simulink model "satellite2"  (R2025b)
settings: Solver=FixedStepAuto  StartTime=0.0  StopTime=5000  FixedStep=dt  MinStep=0.0001  RelTol=1e-3
values from neighbouring files (symbols this model uses):
  A_mw = [ ... (first row only)    [init_params.m]
  A_w = [ ... (first row only)    [init_params.m]
  alpha1 = 0.1    [init_params.m]
  alpha2 = 0.1    [init_params.m]
  angle0 = eAR'    [init_params.m]
  area_d = 4    [init_params.m]
  area_m2 = 0.0127    [init_params.m]
  area_s = 2    [init_params.m]
  ARW_deg_per_sqrt_h = 0.01    [init_params.m]
  B_mw = [ ... (first row only)    [init_params.m]
  beta1 = 0.01    [init_params.m]
  beta2 = 0.01    [init_params.m]
  bias0_deg_h = 0.01    [init_params.m]
  C_bus = 0.001    [init_params.m]
  C_mw = [ ... (first row only)    [init_params.m]
  Cd = 2.2    [init_params.m]
  cos_g_max = cos(gamma_max)    [init_params.m]
  Cr = 1.2    [init_params.m]
  D_max = 1    [init_params.m]
  Delta_D = 0.001    [init_params.m]
  dP_th = 0.05    [init_params.m]
  epsilon = 0.01    [init_params.m]
  eta = 0.7    [init_params.m]
  eta_buck = 0.9    [init_params.m]
  eta_chg = 0.95    [init_params.m]
  f = 2.2e9    (= 2200000000)    [init_params.m]
  f_n_hz = 400    [init_params.m]
  g0 = 9.80665    [init_params.m]
  G0 = 1366.1    [init_params.m]
  Gr_dB = 20    [init_params.m]
  Gt_dB = 3    [init_params.m]
  H = 50e3    (= 50000)    [init_params.m]
  h_ref = 400e3    (= 400000)    [init_params.m]
  hat_s = [1;0;0]    [init_params.m]
  I_chg_max = 8    [init_params.m]
  I_dis_max = 10    [init_params.m]
  I_e = 11    [init_params.m]
  I_gate = 0.5    [init_params.m]
  I_triggle = 8    [init_params.m]
  initial_phase = 0    [init_params.m]
  Isp = 220    [init_params.m]
  Iw = 0.02    [init_params.m]
  J2 = 1.08262668e-3    (= 0.00108262668)    [init_params.m]
  Jx = 10    [init_params.m]
  Jy = 12    [init_params.m]
  Jz = 8    [init_params.m]
  k_a = 4e-4    (= 0.0004)    [init_params.m]
  k_bias1_deg_h_per_C = 1    [init_params.m]
  k_bias2_deg_h_per_C = 0.0    (= 0)    [init_params.m]
  k_sf1_ppm = 1.0    (= 1)    [init_params.m]
  k_sf2_ppm = 0.0    (= 0)    [init_params.m]
  K_w = A_w' / (A_w * A_w')    [init_params.m]
  Kd = [ ... (first row only)    [init_params.m]
  kI = 0.01    [init_params.m]
  Kp = [ ... (first row only)    [init_params.m]
  kP = 10    [init_params.m]
  m = 500    [init_params.m]
  m0 = 20    [init_params.m]
  mu = 3.986004418e14    (= 398600441800000)    [init_params.m]
  n_solar = [1;0;0]    [init_params.m]
  omegaE = 7.2921159e-5    (= 7.2921159e-05)    [init_params.m]
  P0 = 4.56e-6    (= 4.56e-06)    [init_params.m]
  P_adcs = 20    [init_params.m]
  P_base = 50    [init_params.m]
  P_cc = 220/V_bus0    (= 7.85714285714)    [init_params.m]
  P_comm = 40    [init_params.m]
  P_prop = 5    [init_params.m]
  P_trickle = 14/V_bus0    (= 0.5)    [init_params.m]
  perimeter_m = 0.4    [init_params.m]
  Pt_dBW = 10    [init_params.m]
  Q = 20    [init_params.m]
  Q0 = [0.6;0.8;0;0]    [init_params.m]
  r1 = 1e-4    (= 0.0001)    [init_params.m]
  r2 = 1e-4    (= 0.0001)    [init_params.m]
  r_ref = 7.026e6    (= 7026000)    [init_params.m]
  Rb = 0.2    [init_params.m]
  Re = 6378137    [init_params.m]
  rho_ref = 3e-12    [init_params.m]
  rpm_max = 6000    [init_params.m]
  sf_factor = 0.85    [init_params.m]
  sigma1 = 0    [init_params.m]
  sigma2 = 0    [init_params.m]
  SOC0 = 0.6    [init_params.m]
  SOC1 = 0.2    [init_params.m]
  SOC2 = 0.8    [init_params.m]
  SOC_low_adcs = 0.1    [init_params.m]
  SOC_low_comm = 0.2    [init_params.m]
  SOC_low_prop = 0.2    [init_params.m]
  sta_vec = Re * [ ... (first row only)    [init_params.m]
  t_a = 0.1    [init_params.m]
  T_max = 0.05    [init_params.m]
  T_nominal = 20    [init_params.m]
  tau12 = 0.001    [init_params.m]
  tau21 = 0.001    [init_params.m]
  tau_th_s = 200    [init_params.m]
  tau_thr = 0.2    [init_params.m]
  theta12 = 0.005    [init_params.m]
  theta21 = 0.005    [init_params.m]
  V_bus0 = 28    [init_params.m]
  V_center = 50    [init_params.m]
  V_max = 33    [init_params.m]
  V_min = 24    [init_params.m]
  V_oc = num_s*Vmp    [init_params.m]
  v_peak_deg_s = 1.0    (= 1)    [init_params.m]
  V_pzt_max = 100    [init_params.m]
  V_pzt_min = 0    [init_params.m]
  vx0 = 0    [init_params.m]
  vy0 = 7546    [init_params.m]
  vz0 = 0    [init_params.m]
  w0 = [0;0;0]    [init_params.m]
  wavelength_m = 632.8e-9    (= 6.328e-07)    [init_params.m]
  white_rate_std_deg_s = 0    [init_params.m]
  x0 = 7e6    (= 7000000)    [init_params.m]
  y0 = 0    [init_params.m]
  z0 = 0    [init_params.m]
  zeta = 0.01    [init_params.m]
libraries: matrix_library x14, simulink x7, nesl_utility x4, simulink_extras x3, fl_lib x3, ee_lib x1
(part 1 of 2)
settings Model: SimulationMode=accelerator  PauseTimes=13000  Creator=NUAA  LastModifiedBy=NUAA
settings SolverCC: InitialStep=0.0001

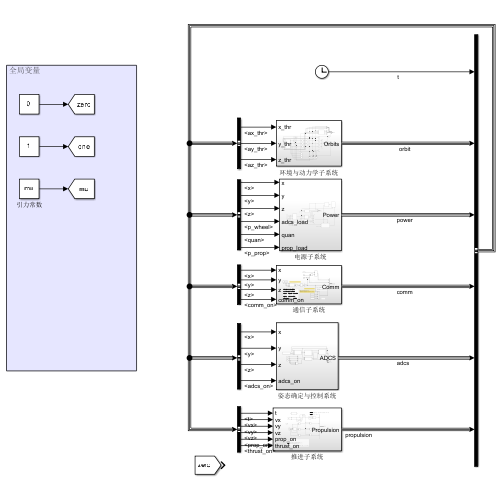
[thumbnail: Simulink's stored preview of the top-level diagram]
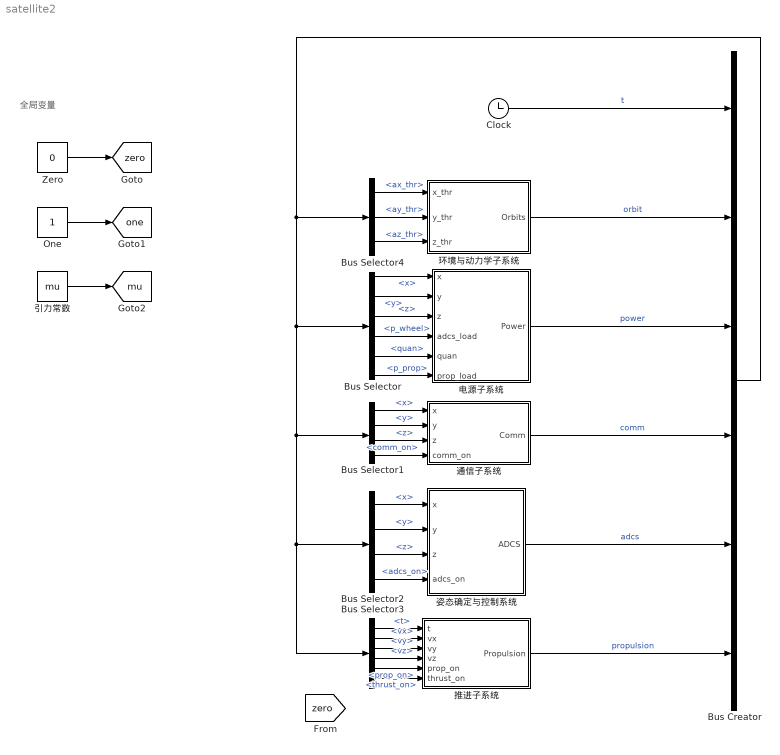
== system satellite2 ==
  note: 全局变量
  Bus Creator : BusCreator  Inputs=6  OutDataTypeStr=Bus: sat
  Bus Selector : BusSelector  OutputSignals=orbit.states.x,orbit.states.y,orbit.states.z,adcs.p_wheel,adcs.quan,propulsion.p_prop
  Bus Selector1 : BusSelector  OutputSignals=orbit.states.x,orbit.states.y,orbit.states.z,power.comm_on
  Bus Selector2 : BusSelector  OutputSignals=orbit.states.x,orbit.states.y,orbit.states.z,power.adcs_on
  Bus Selector3 : BusSelector  OutputSignals=t,orbit.states.vx,orbit.states.vy,orbit.states.vz,power.prop_on,orbit.thrust_on
  Bus Selector4 : BusSelector  OutputSignals=propulsion.ax_thr,propulsion.ay_thr,propulsion.az_thr
  Clock : Clock
  One : Constant  OutDataTypeStr=Inherit: Inherit via back propagation
  Zero : Constant  Value=0  OutDataTypeStr=Inherit: Inherit via back propagation
  姿态确定与控制系统 : Subsystem
  引力常数 : Constant  Value=mu  OutDataTypeStr=Inherit: Inherit via back propagation
  推进子系统 : Subsystem
  环境与动力学子系统 : Subsystem
  电源子系统 : Subsystem
  通信子系统 : Subsystem
  tag scope: mu=global, one=global, zero=global
  wires:
  Zero/1 -> [zero]
  One/1 -> [one]
  引力常数/1 -> [mu]
  环境与动力学子系统/1(Orbits) -> Bus Creator/2  "orbit"
  电源子系统/1(Power) -> Bus Creator/3  "power"
  Bus Creator/1 -> Bus Selector/1, Bus Selector3/1, Bus Selector2/1, Bus Selector1/1, Bus Selector4/1
  通信子系统/1(Comm) -> Bus Creator/4  "comm"
  姿态确定与控制系统/1(ADCS) -> Bus Creator/5  "adcs"
  Bus Selector/1 -> 电源子系统/1(x)  "<x>"
  Bus Selector/3 -> 电源子系统/3(z)  "<z>"
  Bus Selector/2 -> 电源子系统/2(y)  "<y>"
  Bus Selector/4 -> 电源子系统/4(adcs_load)  "<p_wheel>"
  Bus Selector/5 -> 电源子系统/5(quan)  "<quan>"
  Bus Selector1/1 -> 通信子系统/1(x)  "<x>"
  Bus Selector1/2 -> 通信子系统/2(y)  "<y>"
  Bus Selector1/3 -> 通信子系统/3(z)  "<z>"
  Bus Selector1/4 -> 通信子系统/4(comm_on)  "<comm_on>"
  Bus Selector2/1 -> 姿态确定与控制系统/1(x)  "<x>"
  Bus Selector2/2 -> 姿态确定与控制系统/2(y)  "<y>"
  Bus Selector2/3 -> 姿态确定与控制系统/3(z)  "<z>"
  Clock/1 -> Bus Creator/1  "t"
  Bus Selector2/4 -> 姿态确定与控制系统/4(adcs_on)  "<adcs_on>"
  Bus Selector3/1 -> 推进子系统/1(t)  "<t>"
  Bus Selector3/2 -> 推进子系统/2(vx)  "<vx>"
  Bus Selector3/3 -> 推进子系统/3(vy)  "<vy>"
  推进子系统/1(Propulsion) -> Bus Creator/6  "propulsion"
  Bus Selector/6 -> 电源子系统/6(prop_load)  "<p_prop>"
  Bus Selector3/5 -> 推进子系统/5(prop_on)  "<prop_on>"
  Bus Selector4/1 -> 环境与动力学子系统/1(x_thr)  "<ax_thr>"
  Bus Selector4/2 -> 环境与动力学子系统/2(y_thr)  "<ay_thr>"
  Bus Selector3/6 -> 推进子系统/6(thrust_on)  "<thrust_on>"
  Bus Selector3/4 -> 推进子系统/4(vz)  "<vz>"
  Bus Selector4/3 -> 环境与动力学子系统/3(z_thr)  "<az_thr>"

== system satellite2/姿态确定与控制系统 ==
  x : Inport
  y : Inport  Port=2
  z : Inport  Port=3
  adcs_on : Inport  Port=4
  Mux : Mux  Inputs=3
  adcs : BusCreator  Inputs=3  OutDataTypeStr=Bus: adcs
  三轴PD控制器 : Subsystem
  三轴姿态动力学子系统 : Subsystem
  向量模长-r_i : Subsystem
  期望四元数 : Constant  Value=[0;1;0;0]
  重力梯度力矩 : Subsystem
  金字塔反作用轮组件 : Subsystem
  ADCS : Outport
  wires:
  三轴PD控制器/1(指令力矩) -> 金字塔反作用轮组件/1(指令力矩)
  金字塔反作用轮组件/1(实际力矩) -> 三轴姿态动力学子系统/1(实际力矩)
  金字塔反作用轮组件/3(轮功耗) -> adcs/1  "p_wheel"
  期望四元数/1 -> 三轴PD控制器/3(期望四元数)
  三轴姿态动力学子系统/2(角速率) -> 三轴PD控制器/2(实际角速率)
  金字塔反作用轮组件/2(轮角动量) -> 三轴姿态动力学子系统/2(轮角动量)
  Mux/1 -> 重力梯度力矩/2(r_i)
  y/1 -> 向量模长-r_i/2(u1), Mux/2
  x/1 -> 向量模长-r_i/1(u0), Mux/1
  z/1 -> 向量模长-r_i/3(u2), Mux/3
  向量模长-r_i/1(|u|) -> 重力梯度力矩/3(|r_i|)
  重力梯度力矩/1(T_gg) -> 三轴姿态动力学子系统/3(重力梯度力矩)
  adcs/1 -> ADCS/1
  三轴姿态动力学子系统/1(四元数) -> adcs/2, 重力梯度力矩/1(q), 三轴PD控制器/1(实际四元数)  "quan"
  三轴姿态动力学子系统/3(欧拉数) -> adcs/3  "euler_angle"
  adcs_on/1 -> 三轴PD控制器/4(on)

== system satellite2/推进子系统 ==
  note: 化学推进器 ：主要消耗推进剂，电功耗只体现在阀门/控制器，可设很小常数。
      | 电推进器 ：电功耗很大，推力很小。
  note: 1. 接收供电指令和点火指令。
      | 2. 计算实际推力 T_actual 。
      | 3. 根据 Isp 计算推进剂消耗，积分得到剩余推进剂质量 m_prop 。
      | 4. 用 四元数 把机体系推力方向旋转到惯性系，得到 F_ix, F_iy 。
      | 5. 输出推进加速度 a_thr_x, a_thr_y 给现有 Dynamics，并输出 P_thruster 给现有 Power。
  t : Inport
  vx : Inport  Port=2
  vy : Inport  Port=3
  vz : Inport  Port=4
  prop_on : Inport  Port=5
  thrust_on : Inport  Port=6
  Add : Sum
  Bus Creator : BusCreator  Inputs=4  OutDataTypeStr=Bus: propulsion
  Constant : Constant  Value=m-m0
  Divide : Product  Inputs=/*
  Divide1 : Product  Inputs=/*
  Divide2 : Product  Inputs=*/
  Divide3 : Product  Inputs=/*
  Product : Product
  Product1 : Product
  Product2 : Product
  Switch : Switch  Criteria=u2 > Threshold  SaturateOnIntegerOverflow=off  InputSameDT=off
  化推燃料 : Subsystem
  向量模长-v : Subsystem
  电推 : Subsystem
  阀门功耗 : Constant  Value=P_prop
  Propulsion : Outport
  wires:
  prop_on/1 -> 化推燃料/1(prop_on)  "电"
  thrust_on/1 -> 化推燃料/2(thrust_on)  "推"
  vy/1 -> Divide1/2, 向量模长-v/2(u2)
  vx/1 -> Divide/2, 向量模长-v/1(u1)
  向量模长-v/1(|u|) -> Divide3/1, Divide/1, Divide1/1
  Constant/1 -> Add/2
  化推燃料/2(left_fuel) -> Add/1
  Add/1 -> Divide2/2
  化推燃料/1(T_act) -> Divide2/1, Switch/2
  Divide/1 -> Product/2
  Divide2/1 -> Product2/1, Product1/1, Product/1
  Divide1/1 -> Product1/2
  阀门功耗/1 -> Switch/1
  [zero] -> Switch/3
  Switch/1 -> Bus Creator/1  "p_prop"
  Product/1 -> Bus Creator/2  "ax_thr"
  Product1/1 -> Bus Creator/3  "ay_thr"
  Bus Creator/1 -> Propulsion/1
  vz/1 -> Divide3/2, 向量模长-v/3(u3)
  Product2/1 -> Bus Creator/4  "az_thr"
  Divide3/1 -> Product2/2

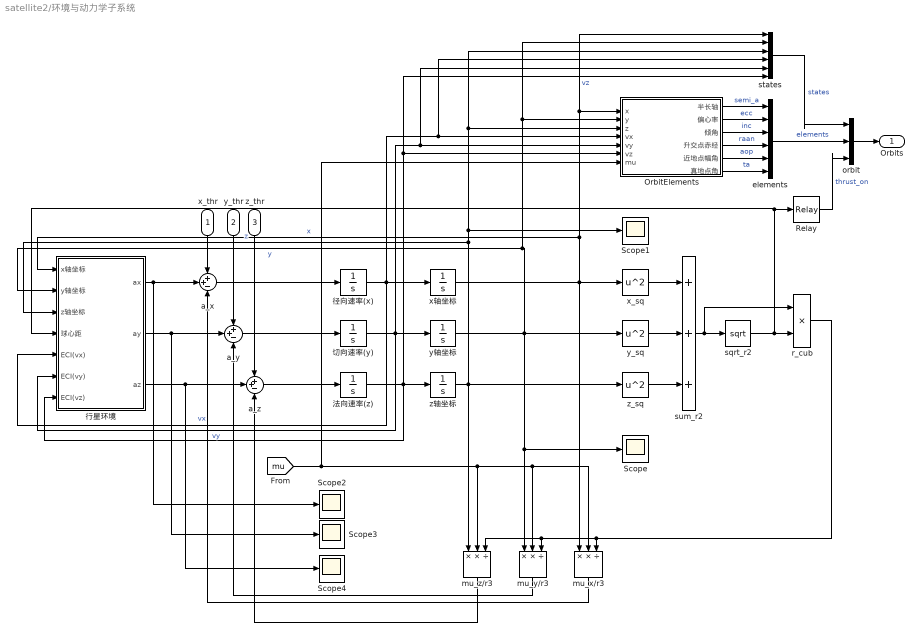
== system satellite2/环境与动力学子系统 ==
  x_thr : Inport
  y_thr : Inport  Port=2
  z_thr : Inport  Port=3
  OrbitElements : Subsystem
  Relay : Relay  OnSwitchValue=r_ref+1e3  OffSwitchValue=r_ref  OnOutputValue=0  OffOutputValue=1  OutDataTypeStr=boolean
  Scope{,1..4} (5 alike) : Scope
      Scope settings: ActiveDisplayYMinimum=-8.7380156946362387E+6  ActiveDisplayYMaximum=8.7381777621754128E+6
      Scope1 settings: ActiveDisplayYMinimum=-1  ActiveDisplayYMaximum=1
      Scope2 settings: ActiveDisplayYMinimum=-0.013724283489942623  ActiveDisplayYMaximum=0.013844629667354235  DataLoggingVariableName=ScopeData2
      Scope3 settings: ActiveDisplayYMinimum=-0.013784437757224171  ActiveDisplayYMaximum=0.013784949077631064  DataLoggingVariableName=ScopeData3
      Scope4 settings: ActiveDisplayYMinimum=-1  ActiveDisplayYMaximum=1  DataLoggingVariableName=ScopeData4
  a_x : Sum  Inputs=++-
  a_y : Sum  Inputs=++-
  a_z : Sum  Inputs=++-
  elements : BusCreator  Inputs=6  OutDataTypeStr=Bus: elements
  mu_x/r3 : Product  Inputs=**/
  mu_y/r3 : Product  Inputs=**/
  mu_z/r3 : Product  Inputs=**/
  orbit : BusCreator  Inputs=3  OutDataTypeStr=Bus: orbit
  r_cub : Product
  sqrt_r2 : Sqrt
  states : BusCreator  Inputs=6  OutDataTypeStr=Bus: states
  sum_r2 : Sum  Inputs=+++
  x_sq : Math  Operator=square
  x轴坐标 : Integrator  InitialCondition=x0
  y_sq : Math  Operator=square
  y轴坐标 : Integrator  InitialCondition=y0
  z_sq : Math  Operator=square
  z轴坐标 : Integrator  InitialCondition=z0
  切向速率(y) : Integrator  InitialCondition=vy0
  径向速率(x) : Integrator  InitialCondition=vx0
  法向速率(z) : Integrator  InitialCondition=vz0
  行星环境 : Subsystem
  Orbits : Outport
  wires:
  径向速率(x)/1 -> states/4, OrbitElements/4(vx), 行星环境/5(ECI(vx)), x轴坐标/1  "vx"
  切向速率(y)/1 -> states/5, OrbitElements/5(vy), 行星环境/6(ECI(vy)), y轴坐标/1  "vy"
  法向速率(z)/1 -> OrbitElements/6(vz), states/6, 行星环境/7(ECI(vz)), z轴坐标/1  "vz"
  y轴坐标/1 -> y_sq/1, states/2, OrbitElements/2(y), 行星环境/2(y轴坐标), mu_y/r3/1, Scope/1  "y"
  x_sq/1 -> sum_r2/1
  y_sq/1 -> sum_r2/2
  z_sq/1 -> sum_r2/3
  sum_r2/1 -> sqrt_r2/1, r_cub/1
  sqrt_r2/1 -> Relay/1, 行星环境/4(球心距), r_cub/2
  [mu] -> OrbitElements/7(mu), mu_x/r3/2, mu_y/r3/2, mu_z/r3/2
  r_cub/1 -> mu_x/r3/3, mu_y/r3/3, mu_z/r3/3
  mu_z/r3/1 -> a_z/3
  a_z/1 -> 法向速率(z)/1
  a_y/1 -> 切向速率(y)/1
  mu_y/r3/1 -> a_y/3
  mu_x/r3/1 -> a_x/3
  x轴坐标/1 -> mu_x/r3/1, x_sq/1, states/1, OrbitElements/1(x), 行星环境/1(x轴坐标)  "x"
  z轴坐标/1 -> z_sq/1, mu_z/r3/1, Scope1/1, states/3, OrbitElements/3(z), 行星环境/3(z轴坐标)  "z"
  行星环境/1(ax) -> a_x/2, Scope2/1
  行星环境/2(ay) -> a_y/2, Scope3/1
  行星环境/3(az) -> a_z/2, Scope4/1
  a_x/1 -> 径向速率(x)/1
  OrbitElements/1(半长轴) -> elements/1  "semi_a"
  OrbitElements/2(偏心率) -> elements/2  "ecc"
  OrbitElements/3(倾角) -> elements/3  "inc"
  OrbitElements/4(升交点赤经) -> elements/4  "raan"
  OrbitElements/5(近地点幅角) -> elements/5  "aop"
  OrbitElements/6(真地点角) -> elements/6  "ta"
  elements/1 -> orbit/2  "elements"
  states/1 -> orbit/1  "states"
  orbit/1 -> Orbits/1
  x_thr/1 -> a_x/1
  y_thr/1 -> a_y/1
  Relay/1 -> orbit/3  "thrust_on"
  z_thr/1 -> a_z/1

== system satellite2/电源子系统 ==
  x : Inport
  y : Inport  Port=2
  z : Inport  Port=3
  adcs_load : Inport  Port=4
  quan : Inport  Port=5
  prop_load : Inport  Port=6
  Add : Sum  Inputs=++++
  power : BusCreator  Inputs=4  OutDataTypeStr=Bus: power
  充放电调节器 : Subsystem
      settings: PortSchema="{\"entries\":[{\"content\":{\"sides\":[{\"content\":{\"connectorIds\":[\"In1\",\"In2\"]},\"type\":\"ConnectorPlacement.EquallySpacedRectSide\",\"uuid\":\"1ee7afef-72a2-44d7-b1fe-f775c1bd2fb5\"},{\"content\":{\"side\":\"RIGHT\"},\"type\":\"ConnectorPlacement.EquallySpacedRectSide\",\"uuid\":\"a705df99-5add-4aef-8a58-2d39c82bf6d7\"},{\"content\":{\"connectorIds\":[\"Out1\"],\"side\":\"TOP\"},\"type\":\"ConnectorPlacement.EquallySpacedRectSide\",\"uuid\":\"759de5c5-d633-4c5d-bf74-673abcd24ad6\"}]},\"type\":\"ConnectorPlacement.EquallySpacedConnector\",\"uuid\":\"7ef34a9a-0568-4899-98ec-73e8b4fd5653\"}],\"packageUris\":[\"http://schema.mathworks.com/mf0/Connector/R2020b\"],\"version\":\"1.0\"}"
  太阳能板 : Subsystem
      settings: PortSchema="{\"entries\":[{\"content\":{\"sides\":[{\"content\":{\"connectorIds\":[\"In1\",\"In2\"]},\"type\":\"ConnectorPlacement.EquallySpacedRectSide\",\"uuid\":\"5bc779c2-c30f-4cae-b4e1-f2edac4125bf\"},{\"content\":{\"connectorIds\":[\"Out1\"],\"side\":\"RIGHT\"},\"type\":\"ConnectorPlacement.EquallySpacedRectSide\",\"uuid\":\"cdc54232-7dcb-45bf-9570-abbf77ba5ff8\"},{\"content\":{\"connectorIds\":[\"In3\",\"In4\"],\"side\":\"TOP\"},\"type\":\"ConnectorPlacement.EquallySpacedRectSide\",\"uuid\":\"7ae4bd94-3445-4ae2-aeac-bc49ea099582\"}]},\"type\":\"ConnectorPlacement.EquallySpacedConnector\",\"uuid\":\"4dec81bf-3de5-48e4-88d8-77ff2b0205f0\"}],\"packageUris\":[\"http://schema.mathworks.com/mf0/Connector/R2020b\"],\"version\":\"1.0\"}"
  姿态确认与控制功耗 : Subsystem
  平台常开负载功耗 : Constant  Value=P_base
  推进子系统功耗 : Subsystem
  日照标志 : Subsystem
  蓄电池组 : Subsystem
      settings: PortSchema="{\"entries\":[{\"content\":{\"sides\":[{\"content\":{},\"type\":\"ConnectorPlacement.EquallySpacedRectSide\",\"uuid\":\"7e7ce6a8-f422-4b44-b417-981bf143e596\"},{\"content\":{\"side\":\"RIGHT\"},\"type\":\"ConnectorPlacement.EquallySpacedRectSide\",\"uuid\":\"32e18879-bd9f-43be-9339-7cab6907b877\"},{\"content\":{\"connectorIds\":[\"Out1\",\"Out2\"],\"side\":\"TOP\"},\"type\":\"ConnectorPlacement.EquallySpacedRectSide\",\"uuid\":\"64b37c81-2d28-4322-9005-45a88751c011\"},{\"content\":{\"connectorIds\":[\"In1\"],\"side\":\"BOTTOM\"},\"type\":\"ConnectorPlacement.EquallySpacedRectSide\",\"uuid\":\"597055be-0b91-4221-a6e9-97960dc29d81\"}]},\"type\":\"ConnectorPlacement.EquallySpacedConnector\",\"uuid\":\"41982541-c784-41b5-be8a-a88d5d627e5c\"}],\"packageUris\":[\"http://schema.mathworks.com/mf0/Connector/R2020b\"],\"version\":\"1.0\"}"
  视线角标志 : Subsystem
  通信子系统功耗 : Subsystem
  Power : Outport
  wires:
  z/1 -> 视线角标志/3(z), 日照标志/3(z)
  x/1 -> 日照标志/1(x), 视线角标志/1(x)
  adcs_load/1 -> 姿态确认与控制功耗/2(adcs_load)
  y/1 -> 视线角标志/2(y), 日照标志/2(y)
  蓄电池组/1(SOC) -> power/1, 推进子系统功耗/1(SOC), 通信子系统功耗/1(SOC), 姿态确认与控制功耗/1(SOC), 充放电调节器/1(荷电状态)  "soc"
  视线角标志/1(Vizlit) -> 通信子系统功耗/2(Vizlit)
  日照标志/1(sunlit) -> 通信子系统功耗/3(sunlit), 太阳能板/1(日照标志)
  充放电调节器/1(净充电电流) -> 蓄电池组/1(净充电电流)
  姿态确认与控制功耗/1(adcs_on) -> power/2  "adcs_on"
  通信子系统功耗/1(comm_on) -> power/3  "comm_on"
  太阳能板/1(蓄电池充电电流) -> 充放电调节器/2(蓄电池充电电流)
  姿态确认与控制功耗/2(P_adcs) -> Add/1
  通信子系统功耗/2(通信功耗) -> Add/2
  Add/1 -> 太阳能板/4(P_load)
  蓄电池组/2(V_batt) -> 太阳能板/3(V_batt)
  power/1 -> Power/1
  quan/1 -> 太阳能板/2(q)
  prop_load/1 -> 推进子系统功耗/2(prop_load)
  平台常开负载功耗/1 -> Add/4
  推进子系统功耗/2(prop_on) -> power/4  "prop_on"
  推进子系统功耗/1(P_prop) -> Add/3

== system satellite2/通信子系统 ==
  note: 通信链可用标志
  note: 接收功率
  note: 信噪比
  note: 把姿态误差引入通信天线增益
      | 引入地面站可见性（地球遮挡）
      | 通信成功 → 数据量积分（任务完成度）
      | 通信失败 → 自动进入安全模式
      | 多地面站切换（Switch + 几何判断）
  note: 如果后面想考虑姿态误差，
      | 只需要在Gt上再减一个pointing loss。
  note: 自由空间路径损耗
      | $\text{FSPL(dB)}=20\log_{10}{(\frac{4\pi r f}{c})}$
  note: 后续可以改成与地面站的距离
  note: 后续可以添加固放和行波管
  x : Inport
  y : Inport  Port=2
  z : Inport  Port=3
  comm_on : Inport  Port=4
  10dB : Constant
  20 : Gain  Gain=20
  4pi rf/c : Gain  Gain=4*pi*f
  > : RelationalOperator  Operator=>  OutDataTypeStr=boolean  RndMeth=Simplest  InputSameDT=off
  AND : Logic  AllPortsSameDT=off  OutDataTypeStr=boolean
  Add : Sum  Inputs=-+++
  Log_10 : Math  Operator=log10
  N_dBW : Constant
  Sum : Sum  Inputs=|-+
  comm : BusCreator  Inputs=4  OutDataTypeStr=Bus: comm
  发射功率 : Constant  Value=Pt_dBW
  向量模长-r : Subsystem
  地面站天线 : Constant  Value=Gr_dB
  星上天线 : Constant  Value=Gt_dB
  Comm : Outport
  wires:
  x/1 -> 向量模长-r/1(u1)
  y/1 -> 向量模长-r/2(u2)
  z/1 -> 向量模长-r/3(u3)
  向量模长-r/1(|u|) -> 4pi rf/c/1
  4pi rf/c/1 -> Log_10/1
  Log_10/1 -> 20/1
  20/1 -> comm/3, Add/1, Sum/2  "FSPL_dB"
  发射功率/1 -> Add/2
  星上天线/1 -> Add/3
  地面站天线/1 -> Add/4
  Add/1 -> comm/4  "Pr_dBW"
  Sum/1 -> comm/2, >/1  "SNR_dB"
  N_dBW/1 -> Sum/1
  10dB/1 -> >/2
  comm_on/1 -> AND/1
  AND/1 -> comm/1  "link_ok"
  >/1 -> AND/2
  comm/1 -> Comm/1

== system satellite2/姿态确定与控制系统/三轴PD控制器 ==
  note: 姿态误差限幅，防止大误差时控制器给出不合理力矩
  实际四元数 : Inport
  实际角速率 : Inport  Port=2
  期望四元数 : Inport  Port=3
  on : Inport  Port=4
  Demux : Demux
  Mux : Mux  Inputs=3
  Product : Product
  Product1 : Product
  Relay(qe0) : Relay  OffOutputValue=-1
  Sum1 : Sum  Inputs=|+-
  sign(q0) : Signum
  共轭-qa^* : Subsystem
  四元数乘法 : Subsystem
  姿态控制器-微分 : Gain  Gain=Kd
  姿态控制器-比例 : Gain  Gain=Kp
  指令力矩 : Outport
  wires:
  Product/1 -> 姿态控制器-比例/1
  姿态控制器-比例/1 -> Sum1/1
  姿态控制器-微分/1 -> Sum1/2
  Product1/1 -> 指令力矩/1
  期望四元数/1 -> 四元数乘法/1(期望)
  实际四元数/1 -> 共轭-qa^*/1(u)
  四元数乘法/1(四元数旋转偏差) -> Demux/1
  Demux/1 -> Relay(qe0)/1
  Demux/2 -> Mux/1
  Demux/3 -> Mux/2
  Demux/4 -> Mux/3
  Mux/1 -> Product/2
  Relay(qe0)/1 -> Product/1
  实际角速率/1 -> 姿态控制器-微分/1
  共轭-qa^*/1(u^-1) -> 四元数乘法/2(实际逆)
  Sum1/1 -> Product1/1
  on/1 -> Product1/2

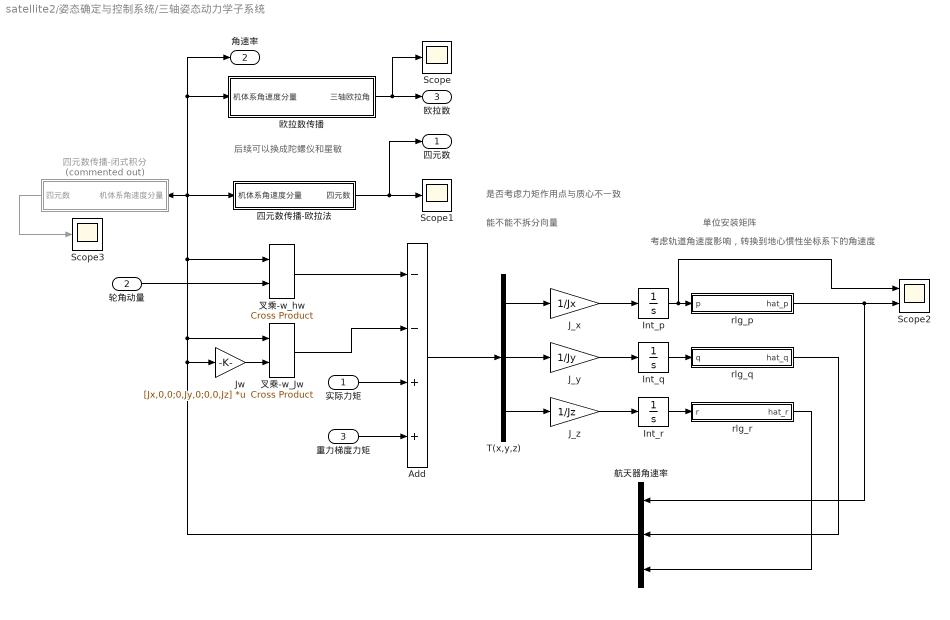
== system satellite2/姿态确定与控制系统/三轴姿态动力学子系统 ==
  note: 考虑轨道角速度影响，转换到地心惯性坐标系下的角速度
  note: 后续可以换成陀螺仪和星敏
  note: 能不能不拆分向量
  note: 是否考虑力矩作用点与质心不一致
  note: 单位安装矩阵
  实际力矩 : Inport
  轮角动量 : Inport  Port=2
  重力梯度力矩 : Inport  Port=3
  Add : Sum  Inputs=--++
  Int_p : Integrator  InitialCondition=w0(1)
  Int_q : Integrator  InitialCondition=w0(1)
  Int_r : Integrator  InitialCondition=w0(3)
  J_x : Gain  Gain=1/Jx
  J_y : Gain  Gain=1/Jy
  J_z : Gain  Gain=1/Jz
  Jw : Gain  Gain=[Jx,0,0;0,Jy,0;0,0,Jz]  Multiplication=Matrix(K*u)
  Scope : Scope
      settings: ActiveDisplayYMinimum=-0.23182380450040346  ActiveDisplayYMaximum=2.0864142405036312  DataLoggingVariableName=ScopeData11
  Scope1 : Scope
      settings: ActiveDisplayYMinimum=-0.13874164124164506  ActiveDisplayYMaximum=1.1265268490250289  DataLoggingVariableName=ScopeData6
  Scope2 : Scope  NumInputPorts=2
      settings: ActiveDisplayYMinimum=0.01821779436387988  ActiveDisplayYMaximum=0.019182857628508503  DataLoggingVariableName=ScopeData6
  Scope3 : Scope
      settings: ActiveDisplayYMinimum=-0.11851103133871327  ActiveDisplayYMaximum=1.0665346715338309  DataLoggingVariableName=ScopeData8
  T(x,y,z) : Demux  Outputs=3
  rlg_p : Subsystem
  rlg_q : Subsystem
  rlg_r : Subsystem
  叉乘-w_Jw : matrix_library/Cross Product
  叉乘-w_hw : matrix_library/Cross Product
  四元数传播-欧拉法 : Subsystem
  四元数传播-闭式积分 : Subsystem  Commented=on
  欧拉数传播 : Subsystem
  航天器角速率 : Mux  Inputs=3
  四元数 : Outport
  角速率 : Outport  Port=2
  欧拉数 : Outport  Port=3
  wires:
  航天器角速率/1 -> 四元数传播-闭式积分/1(机体系角速度分量), 四元数传播-欧拉法/1(机体系角速度分量), 欧拉数传播/1(机体系角速度分量), 角速率/1, 叉乘-w_hw/1, 叉乘-w_Jw/1, Jw/1
  Add/1 -> T(x,y,z)/1
  叉乘-w_hw/1 -> Add/1
  轮角动量/1 -> 叉乘-w_hw/2
  实际力矩/1 -> Add/3
  J_z/1 -> Int_r/1
  T(x,y,z)/1 -> J_x/1
  J_y/1 -> Int_q/1
  T(x,y,z)/2 -> J_y/1
  J_x/1 -> Int_p/1
  T(x,y,z)/3 -> J_z/1
  Int_p/1 -> Scope2/1, rlg_p/1(p)
  Int_q/1 -> rlg_q/1(q)
  Int_r/1 -> rlg_r/1(r)
  Jw/1 -> 叉乘-w_Jw/2
  叉乘-w_Jw/1 -> Add/2
  重力梯度力矩/1 -> Add/4
  rlg_p/1(hat_p) -> 航天器角速率/1, Scope2/2
  rlg_q/1(hat_q) -> 航天器角速率/2
  rlg_r/1(hat_r) -> 航天器角速率/3
  四元数传播-闭式积分/1(四元数) -> Scope3/1
  四元数传播-欧拉法/1(四元数) -> 四元数/1, Scope1/1
  欧拉数传播/1(三轴欧拉角) -> Scope/1, 欧拉数/1

== system satellite2/姿态确定与控制系统/向量模长-r_i ==
  u0 : Inport
  u1 : Inport  Port=2
  u2 : Inport  Port=3
  Add : Sum  Inputs=3
  Sqrt : Sqrt
  Square : Math  Operator=square
  Square1 : Math  Operator=square
  Square2 : Math  Operator=square
  |u| : Outport
  wires:
  u0/1 -> Square/1
  u1/1 -> Square1/1
  u2/1 -> Square2/1
  Square/1 -> Add/1
  Square1/1 -> Add/2
  Square2/1 -> Add/3
  Add/1 -> Sqrt/1
  Sqrt/1 -> |u|/1

== system satellite2/姿态确定与控制系统/重力梯度力矩 ==
  note: $\text{T}_{gg}=3\frac{\mu}{r^3}\hat{r}_B\times (J\hat{r}_B)$
  q : Inport
  r_i : Inport  Port=2
  |r_i| : Inport  Port=3
  Constant : Constant  Value=3
  Divide : Product  Inputs=/*
  Gain : Gain  Gain=3
  Mux : Mux  Inputs=2
  Pow : Math  Operator=pow  OutputSignalType=real  RndMeth=Zero
  Product : Product  Multiplication=Matrix(*)
  Product1 : Product
  hat-r_b : Subsystem
  共轭 : Subsystem
  卫星对角转动惯量 : Constant  Value=[Jx,0,0;0,Jy,0;0,0,Jz]
  叉乘-r_Jr : matrix_library/Cross Product
  四元数乘法 : Subsystem
  T_gg : Outport
  wires:
  [mu] -> Gain/1
  共轭/1(q*) -> 四元数乘法/1(Q1)
  r_i/1 -> Mux/2
  四元数乘法/1(Q*) -> hat-r_b/1(Q1)
  |r_i|/1 -> Pow/1
  Constant/1 -> Pow/2
  卫星对角转动惯量/1 -> Product/1
  hat-r_b/1(Q*) -> Product/2, 叉乘-r_Jr/1
  Product/1 -> 叉乘-r_Jr/2
  Gain/1 -> Divide/2
  Pow/1 -> Divide/1
  Divide/1 -> Product1/2
  叉乘-r_Jr/1 -> Product1/1
  Product1/1 -> T_gg/1
  [zero] -> Mux/1
  Mux/1 -> 四元数乘法/2(Q2)
  q/1 -> hat-r_b/2(Q2), 共轭/1(q)

== system satellite2/姿态确定与控制系统/金字塔反作用轮组件 ==
  note: 后续可以换成双闭环速度伺服系统
  指令力矩 : Inport
  1/eta : Gain  Gain=1/eta
  Abs : Abs  SaturateOnIntegerOverflow=off
  Product : Product
  Relational Operator : RelationalOperator  Operator=>  OutDataTypeStr=boolean  RndMeth=Simplest  InputSameDT=off
  State-Space : StateSpace  A=A_mw  B=B_mw  C=C_mw  D=zeros(4,4)  InitialCondition=0
  Sum of Elements : Sum  Inputs=+
  分配矩阵 : Gain  Gain=K_w  Multiplication=Matrix(K*u)
  力矩限幅 : Saturate  UpperLimit=T_max  LowerLimit=-T_max
  安全转速 : Constant  Value=rpm_max*sf_factor
  安装矩阵 : Gain  Gain=A_w  Multiplication=Matrix(K*u)
  安装矩阵1 : Gain  Gain=A_w  Multiplication=Matrix(K*u)
  转动惯量 : Gain  Gain=Iw
  轮速积分 : Integrator
  除以转动惯量 : Gain  Gain=1/Iw
  实际力矩 : Outport
  轮角动量 : Outport  Port=2
  轮功耗 : Outport  Port=3
  饱和标志 : Outport  Port=4
  wires:
  除以转动惯量/1 -> 轮速积分/1
  State-Space/1 -> 力矩限幅/1
  轮速积分/1 -> Relational Operator/1, 转动惯量/1, Product/2
  Product/1 -> Abs/1
  力矩限幅/1 -> 安装矩阵/1, Product/1, 除以转动惯量/1
  安装矩阵/1 -> 实际力矩/1
  分配矩阵/1 -> State-Space/1
  指令力矩/1 -> 分配矩阵/1
  Abs/1 -> Sum of Elements/1
  Sum of Elements/1 -> 1/eta/1
  1/eta/1 -> 轮功耗/1
  转动惯量/1 -> 安装矩阵1/1
  安装矩阵1/1 -> 轮角动量/1
  安全转速/1 -> Relational Operator/2
  Relational Operator/1 -> 饱和标志/1

== system satellite2/推进子系统/化推燃料 ==
  prop_on : Inport
  thrust_on : Inport  Port=2
  Isp_g0 : Product
  Logical Operator : Logic  Inputs=3  AllPortsSameDT=off  OutDataTypeStr=boolean
  Scope : Scope
      settings: ActiveDisplayYMinimum=-1  ActiveDisplayYMaximum=1  DataLoggingVariableName=ScopeData12
  Transfer Fcn1 : TransferFcn  Denominator=[tau_thr 1]
  div_mdot : Product  Inputs=/*
  left_m : Integrator  InitialCondition=m0
  neg_mdot : Gain  Gain=-1
  sat_m : Saturate  UpperLimit=m0  LowerLimit=0
  推力 : Constant  Value=T_nominal
  比冲 : Constant  Value=Isp
  燃料约束 : RelationalOperator  Operator=>  OutDataTypeStr=boolean  RndMeth=Simplest  InputSameDT=off
  输出推力 : Switch  Criteria=u2 > Threshold  Threshold=0.5  SaturateOnIntegerOverflow=off  InputSameDT=off
  重力加速度 : Constant  Value=g0
  T_act : Outport
  left_fuel : Outport  Port=2
  wires:
  prop_on/1 -> Logical Operator/1  "电"
  thrust_on/1 -> Scope/1, Logical Operator/2  "推"
  neg_mdot/1 -> left_m/1
  Isp_g0/1 -> div_mdot/1
  重力加速度/1 -> Isp_g0/2
  div_mdot/1 -> neg_mdot/1
  Logical Operator/1 -> 输出推力/2
  比冲/1 -> Isp_g0/1
  输出推力/1 -> T_act/1, div_mdot/2  "T_act"
  [zero] -> 燃料约束/2
  left_m/1 -> sat_m/1
  燃料约束/1 -> Logical Operator/3  "油"
  [zero] -> 输出推力/3
  sat_m/1 -> left_fuel/1, 燃料约束/1
  推力/1 -> 输出推力/1

== system satellite2/推进子系统/向量模长-v ==
  u1 : Inport
  u2 : Inport  Port=2
  u3 : Inport  Port=3
  Add : Sum  Inputs=+++
  Sqrt : Sqrt
  Square : Math  Operator=square
  Square1 : Math  Operator=square
  Square2 : Math  Operator=square
  |u| : Outport
  wires:
  u1/1 -> Square/1
  u2/1 -> Square1/1
  u3/1 -> Square2/1
  Square/1 -> Add/1
  Square1/1 -> Add/2
  Square2/1 -> Add/3
  Add/1 -> Sqrt/1
  Sqrt/1 -> |u|/1

== system satellite2/推进子系统/电推 ==
  In1 : Inport
  Out1 : Outport
  wires:
  In1/1 -> Out1/1

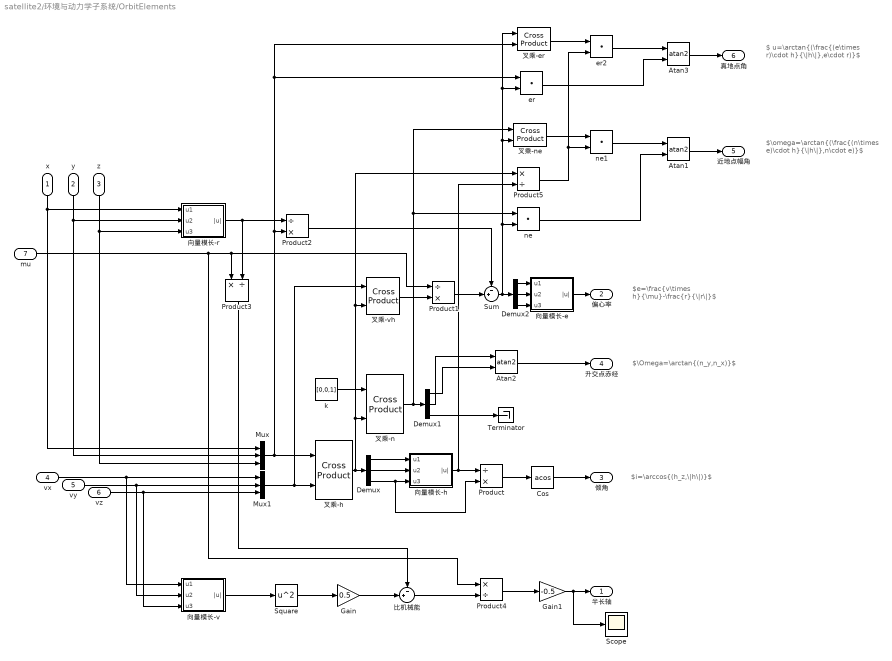
== system satellite2/环境与动力学子系统/OrbitElements ==
  note: $i=\arccos{(h_z,\|h\|)}$
  note: $\Omega=\arctan{(n_y,n_x)}$
  note: $e=\frac{v\times h}{\mu}-\frac{r}{\|r\|}$
  note: $\nu=\arctan{(\frac{(e\times r)\cdot h}{\|h\|},e\cdot r)}$
  note: $\omega=\arctan{(\frac{(n\times e)\cdot h}{\|h\|},n\cdot e)}$
  x : Inport
  y : Inport  Port=2
  z : Inport  Port=3
  vx : Inport  Port=4
  vy : Inport  Port=5
  vz : Inport  Port=6
  mu : Inport  Port=7
  Atan1 : Trigonometry  Operator=atan2
  Atan2 : Trigonometry  Operator=atan2
  Atan3 : Trigonometry  Operator=atan2
  Cos : Trigonometry  Operator=acos
  Demux : Demux  Outputs=3
  Demux1 : Demux  Outputs=3
  Demux2 : Demux  Outputs=3
  Gain : Gain  Gain=0.5
  Gain1 : Gain  Gain=-0.5
  Mux : Mux  Inputs=3
  Mux1 : Mux  Inputs=3
  Product : Product  Inputs=/*
  Product1 : Product  Inputs=/*
  Product2 : Product  Inputs=/*
  Product3 : Product  Inputs=*/
  Product4 : Product  Inputs=*/
  Product5 : Product  Inputs=*/
  Scope : Scope
      settings: ActiveDisplayYMinimum=6.9998946769833127E+6  ActiveDisplayYMaximum=6.9999592468459941E+6  DataLoggingVariableName=ScopeData14
  Square : Math  Operator=square
  Sum : Sum  Inputs=-+|
  Terminator : Terminator
  er : DotProduct  OutDataTypeStr=Inherit: Inherit via internal rule
  er2 : DotProduct  OutDataTypeStr=Inherit: Inherit via internal rule
  k : Constant  Value=[0,0,1]
  ne : DotProduct  OutDataTypeStr=Inherit: Inherit via internal rule
  ne1 : DotProduct  OutDataTypeStr=Inherit: Inherit via internal rule
  叉乘-er : matrix_library/Cross Product
  叉乘-h : matrix_library/Cross Product
  叉乘-n : matrix_library/Cross Product
  叉乘-ne : matrix_library/Cross Product
  叉乘-vh : matrix_library/Cross Product
  向量模长-e : Subsystem
  向量模长-h : Subsystem
  向量模长-r : Subsystem
  向量模长-v : Subsystem
  比机械能 : Sum  Inputs=-+|
  半长轴 : Outport
  偏心率 : Outport  Port=2
  倾角 : Outport  Port=3
  升交点赤经 : Outport  Port=4
  近地点幅角 : Outport  Port=5
  真地点角 : Outport  Port=6
  wires:
  Product/1 -> Cos/1
  向量模长-h/1(|u|) -> Product/1, Product5/2
  Demux/2 -> 向量模长-h/2(u2)
  z/1 -> Mux/3, 向量模长-r/3(u3)
  vx/1 -> Mux1/1, 向量模长-v/1(u1)
  y/1 -> Mux/2, 向量模长-r/2(u2)
  vy/1 -> 向量模长-v/2(u2), Mux1/2
  x/1 -> Mux/1, 向量模长-r/1(u1)
  vz/1 -> Mux1/3, 向量模长-v/3(u3)
  Mux/1 -> er/1, 叉乘-er/2, Product2/2, 叉乘-h/1
  Demux/1 -> 向量模长-h/1(u1)
  Mux1/1 -> 叉乘-h/2, 叉乘-vh/1
  Demux/3 -> Product/2, 向量模长-h/3(u3)
  Cos/1 -> 倾角/1
  叉乘-h/1 -> Product5/1, 叉乘-vh/2, 叉乘-n/2, Demux/1
  叉乘-n/1 -> ne/1, 叉乘-ne/1, Demux1/1
  k/1 -> 叉乘-n/1
  Demux1/1 -> Atan2/2
  Demux1/2 -> Atan2/1
  Demux1/3 -> Terminator/1
  Atan2/1 -> 升交点赤经/1
  叉乘-vh/1 -> Product1/2
  mu/1 -> Product4/1, Product3/1, Product1/1
  向量模长-r/1(|u|) -> Product3/2, Product2/1
  Product1/1 -> Sum/2
  Product2/1 -> Sum/1
  Demux2/1 -> 向量模长-e/1(u1)
  Demux2/2 -> 向量模长-e/2(u2)
  Demux2/3 -> 向量模长-e/3(u3)
  向量模长-e/1(|u|) -> 偏心率/1
  向量模长-v/1(|u|) -> Square/1
  Square/1 -> Gain/1
  Gain/1 -> 比机械能/2
  Product3/1 -> 比机械能/1
  Product4/1 -> Gain1/1
  比机械能/1 -> Product4/2
  Gain1/1 -> Scope/1, 半长轴/1
  叉乘-ne/1 -> ne1/1
  ne1/1 -> Atan1/1
  ne/1 -> Atan1/2
  Atan1/1 -> 近地点幅角/1
  Sum/1 -> ne/2, er/2, 叉乘-er/1, 叉乘-ne/2, Demux2/1
  叉乘-er/1 -> er2/1
  er2/1 -> Atan3/1
  er/1 -> Atan3/2
  Atan3/1 -> 真地点角/1
  Product5/1 -> er2/2, ne1/2

== system satellite2/环境与动力学子系统/行星环境 ==
  x轴坐标 : Inport
  y轴坐标 : Inport  Port=2
  z轴坐标 : Inport  Port=3
  球心距 : Inport  Port=4
  ECI(vx) : Inport  Port=5
  ECI(vy) : Inport  Port=6
  ECI(vz) : Inport  Port=7
  Add : Sum  Inputs=+++
  Add1 : Sum  Inputs=+++
  Add2 : Sum  Inputs=+++
  J2摄动 : Subsystem
  Mux : Mux  Inputs=3
  大气阻力摄动 : Subsystem
  太阳光压摄动 : Subsystem
  ax : Outport
  ay : Outport  Port=2
  az : Outport  Port=3
  wires:
  x轴坐标/1 -> J2摄动/1(x轴坐标), 大气阻力摄动/1(x轴坐标), Mux/1
  y轴坐标/1 -> J2摄动/2(y轴坐标), 大气阻力摄动/2(y轴坐标), Mux/2
  z轴坐标/1 -> J2摄动/3(z轴坐标), Mux/3
  球心距/1 -> 大气阻力摄动/3(球心距), J2摄动/4(球心距)
  ECI(vx)/1 -> 大气阻力摄动/4(径向速率(x))
  ECI(vy)/1 -> 大气阻力摄动/5(切向速率(y))
  ECI(vz)/1 -> 大气阻力摄动/6(法向速率(z))
  J2摄动/1(J2x) -> Add/1
  大气阻力摄动/1(Dx) -> Add/2
  Add/1 -> ax/1
  J2摄动/2(J2y) -> Add1/1
  大气阻力摄动/2(Dy) -> Add1/2
  Add1/1 -> ay/1
  J2摄动/3(J2z) -> Add2/1
  大气阻力摄动/3(Dz) -> Add2/2
  Add2/1 -> az/1
  Mux/1 -> 太阳光压摄动/1(三轴坐标)
  太阳光压摄动/1(srp_x) -> Add/3
  太阳光压摄动/2(srp_y) -> Add1/3
  太阳光压摄动/3(srp_z) -> Add2/3

== system satellite2/电源子系统/充放电调节器 ==
  荷电状态 : Inport
  蓄电池充电电流 : Inport  Port=2
  1-SOC2 : Gain  Gain=1/(1-SOC2)
  Add1 : Sum  Inputs=+-
  Inet_gt_0 : RelationalOperator  Operator=>  OutDataTypeStr=boolean  RndMeth=Simplest  InputSameDT=off
  Inet_gt_Ilimit : RelationalOperator  Operator=<  OutDataTypeStr=boolean  RndMeth=Simplest  InputSameDT=off
  SOC1 : Constant  Value=SOC1
  SOC2 : Constant  Value=SOC2
  SOC_lt_SOC1 : RelationalOperator  Operator=>  OutDataTypeStr=boolean  RndMeth=Simplest  InputSameDT=off
  SOC_lt_SOC2 : RelationalOperator  Operator=>  OutDataTypeStr=boolean  RndMeth=Simplest  InputSameDT=off
  Zero : Constant  Value=0  OutDataTypeStr=Inherit: Inherit via back propagation
  充电|放电 : Switch  Criteria=u2 > Threshold  SaturateOnIntegerOverflow=off  InputSameDT=off
  充电限制|不限制 : Switch  Criteria=u2 > Threshold  SaturateOnIntegerOverflow=off  InputSameDT=off
  涓流|稳流 : Switch  Criteria=u2 > Threshold  SaturateOnIntegerOverflow=off  InputSameDT=off
  涓流充电电流 : Constant  Value=P_trickle
  稳压充电电流 : Product
  稳压充电系数限幅 : Saturate  UpperLimit=1  LowerLimit=0
  稳流|稳压 : Switch  Criteria=u2 > Threshold  SaturateOnIntegerOverflow=off  InputSameDT=off
  稳流充电电流 : Constant  Value=P_cc
  净充电电流 : Outport
  wires:
  [one] -> Add1/1
  蓄电池充电电流/1 -> Inet_gt_Ilimit/2, 充电|放电/3, Inet_gt_0/1, 充电限制|不限制/3
  SOC_lt_SOC2/1 -> 稳流|稳压/2
  稳压充电电流/1 -> 稳流|稳压/3
  Inet_gt_Ilimit/1 -> 充电限制|不限制/2
  荷电状态/1 -> SOC_lt_SOC2/2, SOC_lt_SOC1/2, Add1/2
  稳流充电电流/1 -> 稳压充电电流/2, 稳流|稳压/1
  1-SOC2/1 -> 稳压充电系数限幅/1
  涓流|稳流/1 -> 充电限制|不限制/1, Inet_gt_Ilimit/1
  SOC_lt_SOC1/1 -> 涓流|稳流/2
  充电|放电/1 -> 净充电电流/1  "I_batt"
  Inet_gt_0/1 -> 充电|放电/2
  充电限制|不限制/1 -> 充电|放电/1
  Add1/1 -> 1-SOC2/1
  SOC1/1 -> SOC_lt_SOC1/1
  SOC2/1 -> SOC_lt_SOC2/1
  稳压充电系数限幅/1 -> 稳压充电电流/1
  涓流充电电流/1 -> 涓流|稳流/1
  稳流|稳压/1 -> 涓流|稳流/3
  Zero/1 -> Inet_gt_0/2

== system satellite2/电源子系统/太阳能板 ==
  note: 最简单的光生电流，后续可改为
      | $I_{pannel}=I_{ph}-I_0\left( e^{\frac{V_{pannel}+IR_s}{nV_t}} -1\right)-\frac{V_{pannel}+IR_s}{R_{sh}}$
  日照标志 : Inport
  q : Inport  Port=2
  V_batt : Inport  Port=3
  P_load : Inport  Port=4
  Add2 : Sum  Inputs=+--
  Constant : Constant  Value=0.1
  Gain : Gain  Gain=1/C_bus
  Gain1 : Gain  Gain=1/Rb
  Integrator : Integrator  InitialCondition=V_bus0
  Max : MinMax  Function=max  Inputs=2
  Product3 : Product  Inputs=*/
  Saturation : Saturate  UpperLimit=I_chg_max  LowerLimit=-I_dis_max
  Sum : Sum  Inputs=|-+
  太阳板 : Subsystem
  母线电压 : Saturate  UpperLimit=inf  LowerLimit=0
  蓄电池充电电流 : Outport
  wires:
  P_load/1 -> Product3/1
  太阳板/1(太阳板输出电流) -> Add2/1
  Product3/1 -> Add2/3  "I_load"
  Gain1/1 -> Saturation/1
  Saturation/1 -> 蓄电池充电电流/1, Add2/2  "蓄电池充电电流"
  Add2/1 -> Gain/1
  Gain/1 -> Integrator/1
  Integrator/1 -> 母线电压/1
  Max/1 -> Product3/2, 太阳板/3(母线电压), Sum/2  "V_bus"
  V_batt/1 -> Sum/1
  Sum/1 -> Gain1/1
  q/1 -> 太阳板/1(q)
  日照标志/1 -> 太阳板/2(日照标志)
  母线电压/1 -> Max/1  "V_bus"
  Constant/1 -> Max/2

== system satellite2/电源子系统/姿态确认与控制功耗 ==
  SOC : Inport
  adcs_load : Inport  Port=2
  0.01 : Constant  Commented=on  Value=0.01
  Add2 : Sum
  SOC_adcs_1/0 : Relay  OnSwitchValue=SOC_low_adcs + 0.02  OffSwitchValue=SOC_low_adcs  OutDataTypeStr=boolean
  Switch : Switch  Criteria=u2 > Threshold  Threshold=0.5  SaturateOnIntegerOverflow=off  InputSameDT=off
  T_gt_001 : RelationalOperator  Commented=on  Operator=<=  OutDataTypeStr=boolean  RndMeth=Simplest  InputSameDT=off
  姿态开时负载功耗 : Constant  Value=P_adcs
  adcs_on : Outport
  P_adcs : Outport  Port=2
  wires:
  Switch/1 -> P_adcs/1
  adcs_load/1 -> Add2/1, T_gt_001/2
  SOC_adcs_1/0/1 -> adcs_on/1, Switch/2
  Add2/1 -> Switch/1
  0.01/1 -> T_gt_001/1
  姿态开时负载功耗/1 -> Add2/2
  [zero] -> Switch/3
  T_gt_001/1 -> ?
  SOC/1 -> SOC_adcs_1/0/1

== system satellite2/电源子系统/推进子系统功耗 ==
  SOC : Inport
  prop_load : Inport  Port=2
  SOC_prop_1/0 : Relay  OnSwitchValue=SOC_low_prop + 0.02  OffSwitchValue=SOC_low_prop  OutDataTypeStr=boolean
  Switch : Switch  Criteria=u2 > Threshold  Threshold=0.5  SaturateOnIntegerOverflow=off  InputSameDT=off
  P_prop : Outport
  prop_on : Outport  Port=2
  wires:
  SOC/1 -> SOC_prop_1/0/1
  SOC_prop_1/0/1 -> prop_on/1, Switch/2
  Switch/1 -> P_prop/1
  prop_load/1 -> Switch/1
  [zero] -> Switch/3

== system satellite2/电源子系统/日照标志 ==
  note: 这是假设x方向由地心指向太阳光方向
  x : Inport
  y : Inport  Port=2
  z : Inport  Port=3
  Add1 : Sum
  Sqrt : Sqrt
  Square : Math  Operator=square
  Square1 : Math  Operator=square
  Zero : Constant  Value=0  OutDataTypeStr=Inherit: Inherit via back propagation
  abs_y_lt_Re : RelationalOperator  Operator=<  OutDataTypeStr=boolean  RndMeth=Simplest  InputSameDT=off
  and_sclipse : Logic  AllPortsSameDT=off  OutDataTypeStr=boolean
  not_sunlit : Logic  Operator=NOT  AllPortsSameDT=off  OutDataTypeStr=boolean
  x_lt_0 : RelationalOperator  Operator=<  OutDataTypeStr=boolean  RndMeth=Simplest  InputSameDT=off
  地球半径 : Constant  Value=Re
  sunlit : Outport
  wires:
  and_sclipse/1 -> not_sunlit/1
  abs_y_lt_Re/1 -> and_sclipse/2
  地球半径/1 -> abs_y_lt_Re/2
  Square1/1 -> Add1/2
  Square/1 -> Add1/1
  Sqrt/1 -> abs_y_lt_Re/1
  Add1/1 -> Sqrt/1
  x_lt_0/1 -> and_sclipse/1
  x/1 -> x_lt_0/1
  z/1 -> Square1/1
  y/1 -> Square/1
  not_sunlit/1 -> sunlit/1
  Zero/1 -> x_lt_0/2

== system satellite2/电源子系统/蓄电池组 ==
  净充电电流 : Inport
  Add3 : Sum
  Constant : Constant  Value=V_max-V_min
  Constant1 : Constant  Value=V_min
  DIV_SOC : Gain  Gain=1/(Q*3600)
  Product : Product
  Relay : Relay
  SOC_delay : Memory  InitialCondition=SOC0
  Scope2 : Scope
      settings: ActiveDisplayYMinimum=0.5861532307196704  ActiveDisplayYMaximum=0.72462092352296614  DataLoggingVariableName=ScopeData9
  Switch : Switch  Criteria=u2 > Threshold  SaturateOnIntegerOverflow=off  InputSameDT=off
  int_SOC : Integrator  InitialCondition=SOC0  LimitOutput=on  UpperSaturationLimit=1  LowerSaturationLimit=0
  充电效率 : Gain  Gain=eta_chg
  放电效率 : Gain  Gain=1/eta_chg
  SOC : Outport
  V_batt : Outport  Port=2
  wires:
  净充电电流/1 -> 放电效率/1, 充电效率/1, Relay/1
  Switch/1 -> DIV_SOC/1
  充电效率/1 -> Switch/1
  Relay/1 -> Switch/2
  放电效率/1 -> Switch/3
  SOC_delay/1 -> Product/1, Scope2/1, SOC/1
  DIV_SOC/1 -> int_SOC/1
  int_SOC/1 -> SOC_delay/1
  Product/1 -> Add3/1
  Constant/1 -> Product/2
  Constant1/1 -> Add3/2
  Add3/1 -> V_batt/1

== system satellite2/电源子系统/视线角标志 ==
  x : Inport
  y : Inport  Port=2
  z : Inport  Port=3
  Mux : Mux  Inputs=3
  余弦夹角 : Subsystem
  地面站向量 : Constant  Value=sta_vec
  小于最大视角 : RelationalOperator  OutDataTypeStr=boolean  RndMeth=Simplest  InputSameDT=off
  最大视线角 : Constant  Value=cos_g_max
  Vizlit : Outport
  wires:
  地面站向量/1 -> 余弦夹角/1(u1)
  Mux/1 -> 余弦夹角/2(u2)
  小于最大视角/1 -> Vizlit/1
  最大视线角/1 -> 小于最大视角/2
  余弦夹角/1(cos(γ)) -> 小于最大视角/1
  x/1 -> Mux/1
  y/1 -> Mux/2
  z/1 -> Mux/3

== system satellite2/电源子系统/通信子系统功耗 ==
  SOC : Inport
  Vizlit : Inport  Port=2
  sunlit : Inport  Port=3
  AND1 : Logic  Inputs=3  AllPortsSameDT=off  OutDataTypeStr=boolean
  SOC_comm_1/0 : Relay  OnSwitchValue=SOC_low_comm + 0.02  OffSwitchValue=SOC_low_comm
  Switch : Switch  Criteria=u2 > Threshold  Threshold=0.5  SaturateOnIntegerOverflow=off  InputSameDT=off
  通信开时负载功耗 : Constant  Value=P_comm
  comm_on : Outport
  通信功耗 : Outport  Port=2
  wires:
  AND1/1 -> Switch/2, comm_on/1
  sunlit/1 -> AND1/3
  通信开时负载功耗/1 -> Switch/1
  SOC_comm_1/0/1 -> AND1/1
  Switch/1 -> 通信功耗/1
  SOC/1 -> SOC_comm_1/0/1
  Vizlit/1 -> AND1/2
  [zero] -> Switch/3

== system satellite2/通信子系统/向量模长-r ==
  u1 : Inport
  u2 : Inport  Port=2
  u3 : Inport  Port=3
  Add : Sum  Inputs=+++
  Sqrt : Sqrt
  Square : Math  Operator=square
  Square1 : Math  Operator=square
  Square2 : Math  Operator=square
  |u| : Outport
  wires:
  u1/1 -> Square/1
  u2/1 -> Square1/1
  u3/1 -> Square2/1
  Square/1 -> Add/1
  Square1/1 -> Add/2
  Square2/1 -> Add/3
  Add/1 -> Sqrt/1
  Sqrt/1 -> |u|/1

== system satellite2/姿态确定与控制系统/三轴PD控制器/共轭-qa^* ==
  u : Inport
  -qd1 : Gain  Gain=-1
  -qd2 : Gain  Gain=-1
  -qd3 : Gain  Gain=-1
  Demux : Demux
  Mux : Mux
  u^-1 : Outport
  wires:
  Mux/1 -> u^-1/1
  Demux/1 -> Mux/1
  Demux/2 -> -qd1/1
  -qd1/1 -> Mux/2
  Demux/3 -> -qd2/1
  -qd2/1 -> Mux/3
  Demux/4 -> -qd3/1
  -qd3/1 -> Mux/4
  u/1 -> Demux/1

== system satellite2/姿态确定与控制系统/三轴PD控制器/四元数乘法 ==
  期望 : Inport
  实际逆 : Inport  Port=2
  Add : Sum  Inputs=3
  Cross Product : matrix_library/Cross Product
  Demux : Demux
  Demux1 : Demux
  Dot Product : DotProduct  OutDataTypeStr=Inherit: Inherit via internal rule
  Mux : Mux  Inputs=2
  Mux1 : Mux  Inputs=3
  Mux2 : Mux  Inputs=3
  Product : Product
  Product1 : Product
  Product2 : Product
  Sum : Sum  Inputs=|+-
  四元数旋转偏差 : Outport
  wires:
  期望/1 -> Demux/1
  实际逆/1 -> Demux1/1
  Mux/1 -> 四元数旋转偏差/1
  Product/1 -> Sum/1
  Demux/1 -> Product1/1, Product/1
  Mux1/1 -> Dot Product/1, Cross Product/1, Product2/2
  Demux1/1 -> Product2/1, Product/2
  Mux2/1 -> Cross Product/2, Dot Product/2, Product1/2
  Sum/1 -> Mux/1
  Dot Product/1 -> Sum/2
  Product2/1 -> Add/2
  Product1/1 -> Add/1
  Cross Product/1 -> Add/3
  Add/1 -> Mux/2
  Demux/2 -> Mux1/1
  Demux/3 -> Mux1/2
  Demux/4 -> Mux1/3
  Demux1/2 -> Mux2/1
  Demux1/3 -> Mux2/2
  Demux1/4 -> Mux2/3

== system satellite2/姿态确定与控制系统/三轴姿态动力学子系统/rlg_p ==
  p : Inport
  Lamb激光动力学 : Subsystem
  Sum : Sum  Inputs=+-|
  Terminator : Terminator
  几何参数 : Subsystem
  噪声模型 : Subsystem
  控模与扫模逻辑 : Subsystem
  机械抖动 : Subsystem  Commented=on
  热模型 : Subsystem
  环境温度 : Sin  Amplitude=10  Bias=25  Frequency=(2*pi)/3600  SampleTime=0
  hat_p : Outport
  wires:
  控模与扫模逻辑/1(扫模电压) -> Lamb激光动力学/5(扫模电压)
  Lamb激光动力学/1(相位差变化率) -> 噪声模型/2(相位差变化率)
  热模型/2(温度标度因数) -> Lamb激光动力学/2(温度标度因数)
  噪声模型/1(测量角速度) -> Sum/2, hat_p/1  "测量角速度"
  几何参数/1(标度因数) -> 噪声模型/1(标度因数), 热模型/2(几何标度因数)
  p/1 -> Lamb激光动力学/1(本体角速度), Sum/1  "本体角速度"
  机械抖动/1(抖动角速度) -> Lamb激光动力学/4(抖动角速度)
  热模型/3(温度零偏) -> Lamb激光动力学/3(零偏速率)
  环境温度/1 -> 热模型/1(环境温度-°C)
  Lamb激光动力学/2(光强) -> 控模与扫模逻辑/1(光强)
  Sum/1 -> Terminator/1

== system satellite2/姿态确定与控制系统/三轴姿态动力学子系统/rlg_q ==
  q : Inport
  Lamb激光动力学 : Subsystem
  Sum : Sum  Inputs=+-|
  Terminator : Terminator
  几何参数 : Subsystem
  噪声模型 : Subsystem
  控模与扫模逻辑 : Subsystem
  机械抖动 : Subsystem  Commented=on
  热模型 : Subsystem
  环境温度 : Sin  Amplitude=10  Bias=25  Frequency=(2*pi)/3600  SampleTime=0
  hat_q : Outport
  wires:
  Sum/1 -> Terminator/1
  Lamb激光动力学/2(光强) -> 控模与扫模逻辑/1(光强)
  环境温度/1 -> 热模型/1(环境温度-°C)
  热模型/3(温度零偏) -> Lamb激光动力学/3(零偏速率)
  机械抖动/1(抖动角速度) -> Lamb激光动力学/4(抖动角速度)
  q/1 -> Sum/1, Lamb激光动力学/1(本体角速度)  "本体角速度"
  几何参数/1(标度因数) -> 热模型/2(几何标度因数), 噪声模型/1(标度因数)
  噪声模型/1(测量角速度) -> hat_q/1, Sum/2  "测量角速度"
  热模型/2(温度标度因数) -> Lamb激光动力学/2(温度标度因数)
  Lamb激光动力学/1(相位差变化率) -> 噪声模型/2(相位差变化率)
  控模与扫模逻辑/1(扫模电压) -> Lamb激光动力学/5(扫模电压)

== system satellite2/姿态确定与控制系统/三轴姿态动力学子系统/rlg_r ==
  r : Inport
  Lamb激光动力学 : Subsystem
  Sum : Sum  Inputs=+-|
  Terminator : Terminator
  几何参数 : Subsystem
  噪声模型 : Subsystem
  控模与扫模逻辑 : Subsystem
  机械抖动 : Subsystem  Commented=on
  热模型 : Subsystem
  环境温度 : Sin  Amplitude=10  Bias=25  Frequency=(2*pi)/3600  SampleTime=0
  hat_r : Outport
  wires:
  控模与扫模逻辑/1(扫模电压) -> Lamb激光动力学/5(扫模电压)
  Lamb激光动力学/1(相位差变化率) -> 噪声模型/2(相位差变化率)
  热模型/2(温度标度因数) -> Lamb激光动力学/2(温度标度因数)
  噪声模型/1(测量角速度) -> Sum/2, hat_r/1  "测量角速度"
  几何参数/1(标度因数) -> 噪声模型/1(标度因数), 热模型/2(几何标度因数)
  r/1 -> Lamb激光动力学/1(本体角速度), Sum/1  "本体角速度"
  机械抖动/1(抖动角速度) -> Lamb激光动力学/4(抖动角速度)
  热模型/3(温度零偏) -> Lamb激光动力学/3(零偏速率)
  环境温度/1 -> 热模型/1(环境温度-°C)
  Lamb激光动力学/2(光强) -> 控模与扫模逻辑/1(光强)
  Sum/1 -> Terminator/1

== system satellite2/姿态确定与控制系统/三轴姿态动力学子系统/四元数传播-欧拉法 ==
  note: $\dot{q}=\frac{1}{2} \left[\begin{array}{ccc} -q_1&-q_2&-q_3 \\ q_0&-q_3&q_2\\ q_3&q_0&-q_1\\ -q_2&q_1&q_0 \end{array}\right]\omega$
  机体系角速度分量 : Inport
  Demux : Demux
  Int_q0 : Integrator  InitialCondition=Q0(1)
  Int_q1 : Integrator  InitialCondition=Q0(2)
  Int_q2 : Integrator  InitialCondition=Q0(3)
  Int_q3 : Integrator  InitialCondition=Q0(4)
  Mux : Mux
  Product : Product  Multiplication=Matrix(*)
  Product{1..4} (4 alike) : Product  Inputs=*/
  Transpose : Math  Operator=transpose
  Vector Concatenate : Concatenate  NumInputs=4  Mode=Multidimensional array  ConcatenateDimension=2
  neg1 : Gain  Gain=-1
  neg2 : Gain  Gain=-1
  neg3 : Gain  Gain=-1
  q0_dot : Mux  Inputs=3
  q1_dot : Mux  Inputs=3
  q1_dot1 : Mux  Inputs=3
  q1_dot2 : Mux  Inputs=3
  向量模长-q : Subsystem
  四元数 : Outport
  wires:
  Product/1 -> Demux/1
  neg1/1 -> q0_dot/1, q1_dot1/3
  q1_dot/1 -> Vector Concatenate/2
  neg3/1 -> q1_dot/2, q0_dot/3
  Product4/1 -> neg3/1, Mux/4, q1_dot1/1  "q3"
  Product1/1 -> q1_dot/1, q1_dot1/2, Mux/1, q1_dot2/3  "q0"
  q1_dot1/1 -> Vector Concatenate/3
  Demux/2 -> Int_q1/1
  Product2/1 -> neg1/1, Mux/2, q1_dot2/2  "q1"
  Demux/3 -> Int_q2/1
  neg2/1 -> q1_dot2/1, q0_dot/2
  q1_dot2/1 -> Vector Concatenate/4
  Product3/1 -> neg2/1, Mux/3, q1_dot/3  "q2"
  q0_dot/1 -> Vector Concatenate/1
  Vector Concatenate/1 -> Transpose/1
  Demux/1 -> Int_q0/1
  Demux/4 -> Int_q3/1
  机体系角速度分量/1 -> Product/2
  Transpose/1 -> Product/1
  Int_q0/1 -> Product1/1, 向量模长-q/1(u0)
  Int_q1/1 -> Product2/1, 向量模长-q/2(u1)
  Int_q2/1 -> Product3/1, 向量模长-q/3(u2)
  Int_q3/1 -> Product4/1, 向量模长-q/4(u3)
  向量模长-q/1(|u|) -> Product2/2, Product3/2, Product4/2, Product1/2
  Mux/1 -> 四元数/1

== system satellite2/姿态确定与控制系统/三轴姿态动力学子系统/四元数传播-闭式积分 ==
  机体系角速度分量 : Inport
  Constant : Constant  Value=1/2
  Cos : Trigonometry  Operator=cos
  Display : Display
  Divide : Product  Inputs=*/
  Dot Product : DotProduct  OutDataTypeStr=Inherit: Inherit via internal rule
  Gain : Gain  Gain=1/2
  Mux : Mux  Inputs=2
  Product : Product
  Sin : Trigonometry
  Sqrt : Sqrt
  Switch : Switch  Criteria=u2 > Threshold  Threshold=1e-6  SaturateOnIntegerOverflow=off  InputSameDT=off
  上一时刻四元数 : UnitDelay  InitialCondition=Q0  SampleTime=t_a  HasFrameUpgradeWarning=on
  四元数乘法 : Subsystem
  解算步长 : Gain  Gain=t_a
  四元数 : Outport
  wires:
  机体系角速度分量/1 -> 解算步长/1
  解算步长/1 -> Dot Product/2, Product/2, Dot Product/1
  Dot Product/1 -> Sqrt/1
  Sqrt/1 -> Gain/1, Divide/2, Switch/2
  Gain/1 -> Cos/1, Sin/1
  Sin/1 -> Divide/1
  Divide/1 -> Switch/1
  Constant/1 -> Switch/3
  Switch/1 -> Product/1
  Product/1 -> Mux/2
  Cos/1 -> Mux/1
  Mux/1 -> Display/1, 四元数乘法/2(Q2)
  四元数乘法/1(Q*) -> 四元数/1, 上一时刻四元数/1
  上一时刻四元数/1 -> 四元数乘法/1(Q1)

== system satellite2/姿态确定与控制系统/三轴姿态动力学子系统/欧拉数传播 ==
  机体系角速度分量 : Inport
  Demux : Demux  Outputs=3
  Gain : Gain  Gain=-1
  Int_phi : Integrator  InitialCondition=angle0(1)
  Int_psi : Integrator  InitialCondition=angle0(3)
  Int_theta : Integrator  InitialCondition=angle0(2)
  Mux{,1..3} (4 alike) : Mux  Inputs=3
  Product : Product  Inputs=**/
  Product1 : Product  Inputs=**/
  Product2 : Product  Inputs=*/
  Product3 : Product  Inputs=/*
  Product4 : Product  Multiplication=Matrix(*)
  Sin1 : Trigonometry
  Sin2 : Trigonometry
  Sin3 : Trigonometry  Operator=cos
  Sin4 : Trigonometry  Operator=cos
  Transpose : Math  Operator=transpose
  Vector Concatenate : Concatenate  NumInputs=3  Mode=Multidimensional array  ConcatenateDimension=2
  三轴欧拉角 : Outport
  wires:
  Mux2/1 -> Vector Concatenate/3
  Gain/1 -> Mux1/3
  Demux/1 -> Int_phi/1
  [one] -> Mux/1
  Demux/3 -> Int_psi/1
  Demux/2 -> Int_theta/1
  Int_psi/1 -> Mux3/3, Sin4/1, Sin2/1  "psi"
  Sin1/1 -> Product/1, Product1/2
  Product1/1 -> Mux/3
  Sin4/1 -> Product3/2, Mux1/2, Product1/1
  Int_theta/1 -> Mux3/2, Sin3/1, Sin1/1  "theta"
  Sin2/1 -> Product/2, Gain/1, Product2/1
  Mux/1 -> Vector Concatenate/1
  Sin3/1 -> Product/3, Product1/3, Product2/2, Product3/1
  Mux1/1 -> Vector Concatenate/2
  Product3/1 -> Mux2/3
  Vector Concatenate/1 -> Transpose/1
  Product2/1 -> Mux2/2
  [zero] -> Mux2/1, Mux1/1
  机体系角速度分量/1 -> Product4/2
  Product/1 -> Mux/2
  Product4/1 -> Demux/1
  Int_phi/1 -> Mux3/1  "phi"
  Transpose/1 -> Product4/1
  Mux3/1 -> 三轴欧拉角/1

== system satellite2/姿态确定与控制系统/重力梯度力矩/hat-r_b ==
  Q1 : Inport
  Q2 : Inport  Port=2
  Add : Sum  Inputs=3
  Cross Product : matrix_library/Cross Product
  Demux : Demux
  Demux1 : Demux
  Demux2 : Demux  Outputs=3
  Divide : Product  Inputs=*/
  Mux1 : Mux  Inputs=3
  Mux2 : Mux  Inputs=3
  Product1 : Product
  Product2 : Product
  向量模长-r_i : Subsystem
  Q* : Outport
  wires:
  Demux1/4 -> Mux2/3
  Demux1/3 -> Mux2/2
  Demux1/2 -> Mux2/1
  Demux/4 -> Mux1/3
  Demux/3 -> Mux1/2
  Demux/2 -> Mux1/1
  Add/1 -> Divide/1, Demux2/1
  Cross Product/1 -> Add/3
  Product1/1 -> Add/1
  Product2/1 -> Add/2
  Mux2/1 -> Product1/2, Cross Product/2
  Demux1/1 -> Product2/1
  Mux1/1 -> Product2/2, Cross Product/1
  Demux/1 -> Product1/1
  Q2/1 -> Demux1/1
  Q1/1 -> Demux/1
  Demux2/1 -> 向量模长-r_i/1(u0)
  Demux2/2 -> 向量模长-r_i/2(u1)
  Demux2/3 -> 向量模长-r_i/3(u2)
  向量模长-r_i/1(|u|) -> Divide/2
  Divide/1 -> Q*/1

== system satellite2/姿态确定与控制系统/重力梯度力矩/共轭 ==
  q : Inport
  -qd1 : Gain  Gain=-1
  -qd2 : Gain  Gain=-1
  -qd3 : Gain  Gain=-1
  Demux : Demux
  Mux : Mux
  q* : Outport
  wires:
  q/1 -> Demux/1
  Mux/1 -> q*/1
  Demux/1 -> Mux/1
  Demux/2 -> -qd1/1
  -qd1/1 -> Mux/2
  Demux/3 -> -qd2/1
  -qd2/1 -> Mux/3
  Demux/4 -> -qd3/1
  -qd3/1 -> Mux/4

== system satellite2/姿态确定与控制系统/重力梯度力矩/四元数乘法 ==
  Q1 : Inport
  Q2 : Inport  Port=2
  Add : Sum  Inputs=3
  Cross Product : matrix_library/Cross Product
  Demux : Demux
  Demux1 : Demux
  Dot Product : DotProduct  OutDataTypeStr=Inherit: Inherit via internal rule
  Mux : Mux  Inputs=2
  Mux1 : Mux  Inputs=3
  Mux2 : Mux  Inputs=3
  Product : Product
  Product1 : Product
  Product2 : Product
  Sum : Sum  Inputs=|+-
  Q* : Outport
  wires:
  Q1/1 -> Demux/1
  Q2/1 -> Demux1/1
  Mux/1 -> Q*/1
  Product/1 -> Sum/1
  Demux/1 -> Product1/1, Product/1
  Mux1/1 -> Dot Product/1, Cross Product/1, Product2/2
  Demux1/1 -> Product2/1, Product/2
  Mux2/1 -> Cross Product/2, Dot Product/2, Product1/2
  Sum/1 -> Mux/1
  Dot Product/1 -> Sum/2
  Product2/1 -> Add/2
  Product1/1 -> Add/1
  Cross Product/1 -> Add/3
  Add/1 -> Mux/2
  Demux/2 -> Mux1/1
  Demux/3 -> Mux1/2
  Demux/4 -> Mux1/3
  Demux1/2 -> Mux2/1
  Demux1/3 -> Mux2/2
  Demux1/4 -> Mux2/3

== system satellite2/环境与动力学子系统/OrbitElements/向量模长-e ==
  u1 : Inport
  u2 : Inport  Port=2
  u3 : Inport  Port=3
  Add : Sum  Inputs=+++
  Sqrt : Sqrt
  Square : Math  Operator=square
  Square1 : Math  Operator=square
  Square2 : Math  Operator=square
  |u| : Outport
  wires:
  u1/1 -> Square/1
  u2/1 -> Square1/1
  u3/1 -> Square2/1
  Square/1 -> Add/1
  Square1/1 -> Add/2
  Square2/1 -> Add/3
  Add/1 -> Sqrt/1
  Sqrt/1 -> |u|/1

== system satellite2/环境与动力学子系统/OrbitElements/向量模长-h ==
  u1 : Inport
  u2 : Inport  Port=2
  u3 : Inport  Port=3
  Add : Sum  Inputs=+++
  Sqrt : Sqrt
  Square : Math  Operator=square
  Square1 : Math  Operator=square
  Square2 : Math  Operator=square
  |u| : Outport
  wires:
  Sqrt/1 -> |u|/1
  Add/1 -> Sqrt/1
  Square2/1 -> Add/3
  Square1/1 -> Add/2
  Square/1 -> Add/1
  u3/1 -> Square2/1
  u2/1 -> Square1/1
  u1/1 -> Square/1

== system satellite2/环境与动力学子系统/OrbitElements/向量模长-r ==
  u1 : Inport
  u2 : Inport  Port=2
  u3 : Inport  Port=3
  Add : Sum  Inputs=+++
  Sqrt : Sqrt
  Square : Math  Operator=square
  Square1 : Math  Operator=square
  Square2 : Math  Operator=square
  |u| : Outport
  wires:
  u1/1 -> Square/1
  u2/1 -> Square1/1
  u3/1 -> Square2/1
  Square/1 -> Add/1
  Square1/1 -> Add/2
  Square2/1 -> Add/3
  Add/1 -> Sqrt/1
  Sqrt/1 -> |u|/1

== system satellite2/环境与动力学子系统/OrbitElements/向量模长-v ==
  u1 : Inport
  u2 : Inport  Port=2
  u3 : Inport  Port=3
  Add : Sum  Inputs=+++
  Sqrt : Sqrt
  Square : Math  Operator=square
  Square1 : Math  Operator=square
  Square2 : Math  Operator=square
  |u| : Outport
  wires:
  Sqrt/1 -> |u|/1
  Add/1 -> Sqrt/1
  Square2/1 -> Add/3
  Square1/1 -> Add/2
  Square/1 -> Add/1
  u3/1 -> Square2/1
  u2/1 -> Square1/1
  u1/1 -> Square/1
